simulink model "model1_11_full"  (R2018a)
settings: Solver=FixedStepAuto  StartTime=0.0  StopTime=31  FixedStep=1e-2  RelTol=1e-3
model workspace (MAT data in the model file):
  J = 0.2
  Ke = 0.19
  Km = 0.2613
  L = 0.048
  N = 62.55
  R = 1.6
  f = 0.02
libraries: simulink x2
settings Model: Creator=0782  LastModifiedBy=0782
settings DataIOCC: ReturnWorkspaceOutputs=on
settings SFSimCC: SimUseLocalCustomCode=on
settings RTWCC: RTWUseLocalCustomCode=on

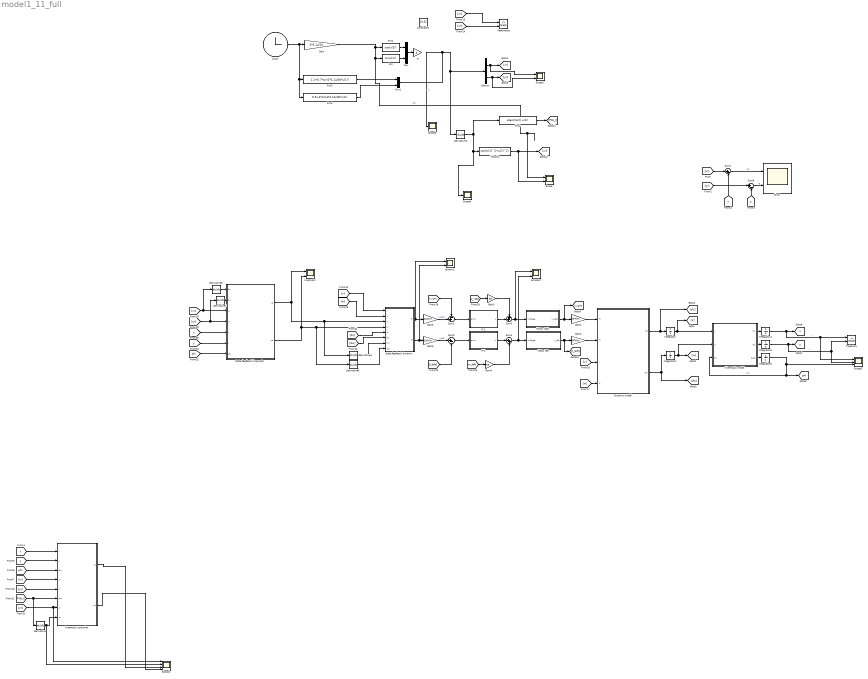
== system model1_11_full ==
  Clock : Clock
  Constant3 : Constant  Value=[3;3]  VectorParams1D=off
  Demux : Demux  Outputs=2
  Derivative{,1,4..7} (6 alike) : Derivative
  Dynamic model : MATLAB Function  TreatAsAtomicUnit=on
  Error : Scope  NumInputPorts=2
  Fcn : Fcn  Expr=sin(u(1))
  Fcn1 : Fcn  Expr=cos(u(1))
  Fcn2 : Fcn  Expr=1.1+0.7*sin(2*3.14/30*u(1))
  Fcn3 : Fcn  Expr=0.9+2*sin(4*3.14/30*u(1))
  Fcn4 : Fcn  Expr=atan2(u(2),u(1))
  Gain : Gain  Gain=2*3.14/10
  Gain1 : Gain  Gain=N*Km
  Gain2 : Gain  Gain=N*Km
  Gain3 : Gain  Gain=Ke
  Gain4 : Gain  Gain=Ke
  Gain5 : Gain  Gain=1/N/Km
  Gain6 : Gain  Gain=1/N/Km
  Integrator : Integrator
  Integrator1 : Integrator
  Integrator4 : Integrator  ContinuousStateAttributes='x'
  Integrator5 : Integrator  ContinuousStateAttributes='y'
  Integrator6 : Integrator  WrapState=on
  Kinematic model : MATLAB Function  TreatAsAtomicUnit=on
  Motor left : Subsystem
  Motor right : Subsystem
  Mux : Mux  Inputs=2
  Mux1 : Mux  Inputs=2
  PI 1 : Subsystem
  PI 2 : Subsystem
  R : Gain  Gain=4
  Referrence : simulink/Sinks/XY Graph  xmin=-3  xmax=3  ymin=-3  ymax=3  st=0.1
  Scope : Scope  NumInputPorts=2
  Scope1 : Scope  NumInputPorts=4
  Scope2 : Scope  NumInputPorts=2
  Scope3 : Scope  NumInputPorts=3
  Scope4 : Scope
  Scope5 : Scope
  State feedback dynamic : MATLAB Function  TreatAsAtomicUnit=on
  State feedback kinematic : MATLAB Function  TreatAsAtomicUnit=on
  Sum1 : Sum  Inputs=|+-
  Sum2 : Sum  Inputs=-+|
  Sum3 : Sum  Inputs=++|
  Sum4 : Sum  Inputs=|++
  Sum5 : Sum  Inputs=|+-
  Sum6 : Sum  Inputs=|+-
  Trajectory : simulink/Sinks/XY Graph  xmin=-3  xmax=3  ymin=-3  ymax=3  st=-1
  Velocity : Fcn  Expr=sqrt(u(1)^2+u(2)^2)
  actuator : Scope  NumInputPorts=2
  dynamic : Scope  NumInputPorts=2
  kinematic : Scope  NumInputPorts=2
  kinematic controller : MATLAB Function  TreatAsAtomicUnit=on
  tag scope: phi=global, x=global, y=global
  wires:
  Integrator1/1 -> Kinematic model/2(w), [w]
  Integrator/1 -> Kinematic model/1(v), [v]
  Dynamic model/1(Dv) -> [dv], Integrator/1
  [v] -> Dynamic model/3(v)
  [w] -> Dynamic model/4(w)
  Motor right/1(I_right) -> [I_right], Gain1/1
  Motor left/1(I_left) -> [I_left], Gain2/1
  Gain1/1 -> Dynamic model/1(Tr)
  Gain2/1 -> Dynamic model/2(Tl)
  Dynamic model/2(Dw) -> Integrator1/1, [dw]
  Integrator5/1 -> Trajectory/2, Scope3/2, [y]  "y"
  Integrator6/1 -> [phi], Kinematic model/3(phi), Scope3/3  "phi"
  Integrator4/1 -> Trajectory/1, Scope3/1, [x]  "x"
  Kinematic model/2(Dy) -> Integrator5/1
  Kinematic model/3(Dphi) -> Integrator6/1
  Kinematic model/1(Dx) -> Integrator4/1
  Sum2/1 -> PI 1/1(error)
  Gain3/1 -> Sum3/1
  [w_right] -> Gain3/1
  PI 1/1(u) -> Sum3/2
  Sum3/1 -> actuator/1, Motor right/1(Voltage)
  [w_left] -> Gain4/1
  Gain4/1 -> Sum4/2
  PI 2/1(u) -> Sum4/1
  Sum4/1 -> actuator/2, Motor left/1(Voltage)
  Sum5/1 -> PI 2/1(error)
  [I_right] -> Sum2/1
  [I_left] -> Sum5/2
  kinematic controller/2(wc) -> Scope1/4
  Derivative5/1 -> State feedback dynamic/8(dwr)
  [dv] -> State feedback dynamic/5(dv)
  [v] -> State feedback dynamic/1(v)
  Derivative4/1 -> State feedback dynamic/7(dvr)
  kinematic controller/1(vc) -> Scope1/3
  [w] -> State feedback dynamic/2(w)
  [dw] -> State feedback dynamic/6(dw)
  State feedback dynamic/1(Tr) -> dynamic/1, Gain5/1
  State feedback dynamic/2(Tl) -> dynamic/2, Gain6/1
  Gain5/1 -> Sum2/2  "I_right"
  Gain6/1 -> Sum5/1  "I_left"
  [phi] -> State feedback kinematic/7(phi)
  Derivative7/1 -> State feedback kinematic/2(dyr)
  [xr] -> Derivative6/1, State feedback kinematic/3(xr)
  Derivative6/1 -> State feedback kinematic/1(dxr)
  [x] -> State feedback kinematic/5(x)
  [y] -> State feedback kinematic/6(y)
  [yr] -> Derivative7/1, State feedback kinematic/4(yr)
  Fcn4/1 -> [PHI_r]
  Fcn3/1 -> Mux1/2
  Derivative1/1 -> Fcn4/1, Scope4/1, Velocity/1
  Fcn2/1 -> Mux1/1
  Clock/1 -> Fcn3/1, Fcn2/1, Gain/1
  Velocity/1 -> Scope/2, [vr]
  [yr] -> Referrence/2
  Fcn/1 -> Mux/2
  [xr] -> Referrence/1
  Mux/1 -> R/1
  Demux/2 -> Scope2/2, [yr]
  Fcn1/1 -> Mux/1
  Demux/1 -> Scope2/1, [xr]
  Gain/1 -> Scope/1, Fcn/1, Fcn1/1  "phi"
  Mux1/1 -> Scope5/1, Derivative1/1, Demux/1  "xy"
  Sum1/1 -> Error/1  "Xe"
  Sum6/1 -> Error/2  "Ye"
  [xr] -> Sum1/1
  [yr] -> Sum6/1
  [x] -> Sum1/2
  [y] -> Sum6/2
  [phi] -> kinematic controller/3(phi)
  Derivative/1 -> Scope1/2, kinematic controller/8(wr)
  [y] -> kinematic controller/2(y)
  [x] -> kinematic controller/1(x)
  [xr] -> kinematic controller/4(xr)
  [vr] -> Scope1/1, kinematic controller/7(vr)
  [yr] -> kinematic controller/5(yr)
  [PHI_r] -> Derivative/1, kinematic controller/6(phir)
  State feedback kinematic/1(vd) -> Derivative4/1, State feedback dynamic/3(vr), kinematic/1
  State feedback kinematic/2(wd) -> kinematic/2, Derivative5/1, State feedback dynamic/4(wr)

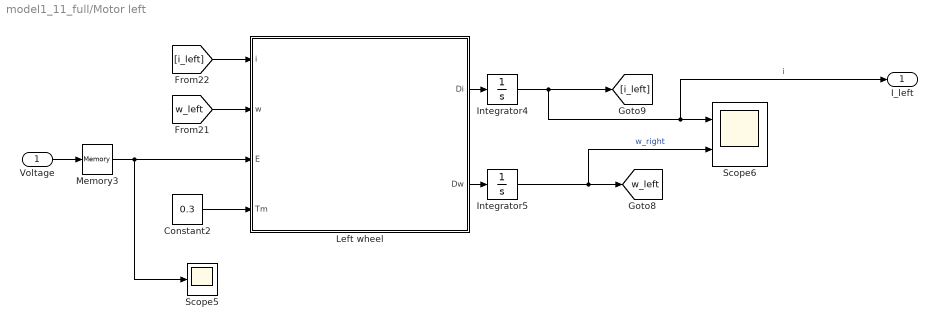
== system model1_11_full/Motor left ==
  Voltage : Inport
  Constant2 : Constant  Value=0.3
  Integrator4 : Integrator
  Integrator5 : Integrator
  Left wheel : MATLAB Function  TreatAsAtomicUnit=on
  Memory3 : Memory
  Scope5 : Scope
  Scope6 : Scope  NumInputPorts=2
  I_left : Outport
  tag scope: w_left=global
  wires:
  Memory3/1 -> Scope5/1, Left wheel/3(E)
  Integrator5/1 -> Scope6/2, [w_left]  "w_right"
  [i_left] -> Left wheel/1(i)
  Left wheel/2(Dw) -> Integrator5/1
  Constant2/1 -> Left wheel/4(Tm)
  [w_left] -> Left wheel/2(w)
  Voltage/1 -> Memory3/1
  Left wheel/1(Di) -> Integrator4/1
  Integrator4/1 -> I_left/1, Scope6/1, [i_left]  "i"

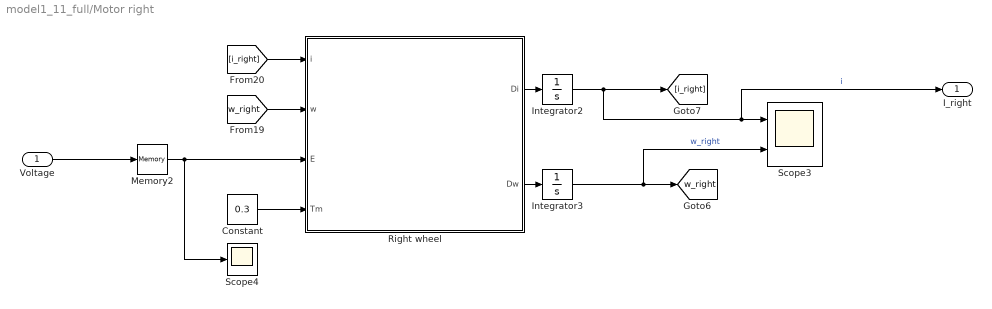
== system model1_11_full/Motor right ==
  Voltage : Inport
  Constant : Constant  Value=0.3
  Integrator2 : Integrator
  Integrator3 : Integrator
  Memory2 : Memory
  Right wheel : MATLAB Function  TreatAsAtomicUnit=on
  Scope3 : Scope  NumInputPorts=2
  Scope4 : Scope
  I_right : Outport
  tag scope: w_right=global
  wires:
  Right wheel/1(Di) -> Integrator2/1
  Integrator3/1 -> Scope3/2, [w_right]  "w_right"
  Constant/1 -> Right wheel/4(Tm)
  [i_right] -> Right wheel/1(i)
  Voltage/1 -> Memory2/1
  [w_right] -> Right wheel/2(w)
  Integrator2/1 -> I_right/1, Scope3/1, [i_right]  "i"
  Right wheel/2(Dw) -> Integrator3/1
  Memory2/1 -> Scope4/1, Right wheel/3(E)

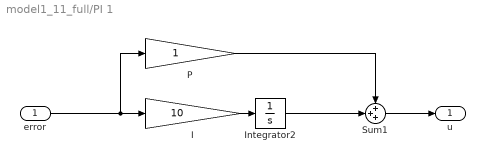
== system model1_11_full/PI 1 ==
  error : Inport
  I : Gain  Gain=10
  Integrator2 : Integrator
  P : Gain
  Sum1 : Sum  Inputs=+++
  u : Outport
  wires:
  error/1 -> P/1, I/1
  I/1 -> Integrator2/1
  P/1 -> Sum1/1
  Integrator2/1 -> Sum1/2
  Sum1/1 -> u/1

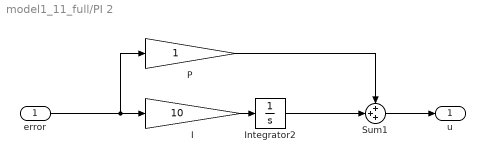
== system model1_11_full/PI 2 ==
  error : Inport
  I : Gain  Gain=10
  Integrator2 : Integrator
  P : Gain
  Sum1 : Sum  Inputs=+++
  u : Outport
  wires:
  error/1 -> P/1, I/1
  I/1 -> Integrator2/1
  P/1 -> Sum1/1
  Integrator2/1 -> Sum1/2
  Sum1/1 -> u/1

== matlab function model1_11_full/kinematic controller ==
  data: x input; vc output; y input; phi input; xr input; yr input; phir input; vr input; wc output; wr input
function [vc,wc] = fcn(x,y,phi,xr,yr,phir,vr,wr)
Kx = 0.001; Ky = .01; Kphi = 0.0001;

xe = xr - x;
ye = yr - y;
phie = phir - phi;

vc = vr*cos(phie) + Kx*xe;
wc = wr + vr*(Ky*ye + Kphi*sin(phie));

== matlab function model1_11_full/Dynamic model ==
  data: Tr input; Dv output size=1; Tl input; Dw output size=1; v input; w input
function [Dv,Dw] = fcn(Tr,Tl,v,w)
mc = 30; Ic = 15.625; R = 0.15; L = 0.375;
d = 0.3; Iw = 0.005; Im = 0.0025; mw = 1;


I = Ic + mc*d^2 + 2*mw*L^2 + 2*Im;
m = mc + 2*mw;

Dv = ((Tr+Tl)/R  + mc*d*w^2)/(m + 2*Iw/R^2);
Dw = ((Tr-Tl)*L/R- mc*d*w*v)/(I + 2*(L/R)^2*Iw);
end

== matlab function model1_11_full/Motor right/Right wheel ==
  data: i input; w input; Di output size=1; E input; Tm input; Dw output size=1; R parameter; Ke parameter; Km parameter; J parameter; f parameter; L parameter
function [Di,Dw] = fcn(i,w,E,Tm,R, Ke, Km, J, f,L)
Di = (E-R*i-Ke*w)/L;
Dw = (Tm - f*w -Km*i)/J;
end

== matlab function model1_11_full/Motor left/Left wheel ==
  data: i input; w input; Di output size=1; E input; Tm input; Dw output size=1; R parameter; Ke parameter; Km parameter; J parameter; f parameter; L parameter
function [Di,Dw] = fcn(i,w,E,Tm,R, Ke, Km, J, f,L)
Di = (E-R*i-Ke*w)/L;
Dw = (Tm - f*w -Km*i)/J;
end

== matlab function model1_11_full/Kinematic model ==
  data: v input size=1; Dx output size=1; w input size=1; phi input size=1; Dy output size=1; Dphi output size=1
function [Dx,Dy,Dphi] = fcn(v,w,phi)

d = 0.3;
Dx = v*cos(phi) - d*w*sin(phi);
Dy = v*sin(phi) + d*w*cos(phi);
Dphi = w;
%{
Dx = v*cos(phi);
Dy = v*sin(phi);
Dphi = w;
%}
end

== matlab function model1_11_full/State feedback dynamic ==
  data: v input; Tr output size=1; w input; vr input; wr input; dv input; dw input; dvr input; dwr input; Tl output size=1
function [Tr,Tl] = fcn(v,w,vr,wr,dv,dw,dvr,dwr)
mc = 30; Ic = 15.625; R = 0.15; L = 0.375;
d = 0.3; Iw = 0.005; Im = 0.0025; mw = 1;
I = Ic + mc*d^2 + 2*mw*L^2 + 2*Im;
m = mc + 2*mw;

Kv = 25; Kw = 25;

Ev = vr - v;
Ew = wr - w;

a = R  * ((dvr + Kv*Ev)*(m + 2*Iw/R^2)     - mc*d*w^2);
b = R/L* ((dwr + Kw*Ew)*(I + 2*L^2*Iw/R^2) + mc*d*w*v);

Tr = (a + b)/2;
Tl = (a - b)/2;
end

== matlab function model1_11_full/State feedback kinematic ==
  data: dxr input; vd output; dyr input; xr input; yr input; x input; y input; phi input; wd output
function [vd,wd] = fcn(dxr,dyr,xr,yr,x,y,phi)
d = 0.3; Kx = 1; Ky = 1;

Ex = xr - x;
Ey = yr - y;

V = [cos(phi), sin(phi);...
    -sin(phi)/d, cos(phi)/d] *([dxr;dyr] + diag([Kx,Ky])*[Ex;Ey]);
vd = V(1);
wd = V(2);

end
